simulink model "Differential_polar_nrz"  (R2020b)
settings: Solver=VariableStepAuto  StartTime=0.0  StopTime=20.0  RelTol=1e-3
libraries: commrandsrc3 x1
settings Model: Creator=mluser  LastModifiedBy=mluser

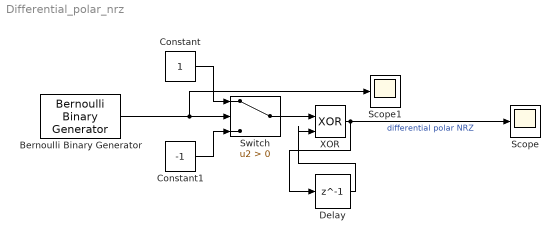
== system Differential_polar_nrz ==
  Bernoulli Binary Generator : commrandsrc3/Bernoulli Binary Generator  ProbabilityOfZero=0.5  SeedSource=Auto  Seed=0  SampleTime=1  SamplesPerFrame=1  OutputDataType=double  SimulateUsing=Interpreted execution
  Constant : Constant
  Constant1 : Constant  Value=-1
  Delay : Delay  DelayLength=1
  Scope : Scope
  Scope1 : Scope
  Switch : Switch  Criteria=u2 > Threshold
  XOR : Logic  Operator=XOR  IconShape=distinctive  AllPortsSameDT=off  OutDataTypeStr=boolean
  wires:
  XOR/1 -> Delay/1, Scope/1  "differential polar NRZ"
  Delay/1 -> XOR/2
  Bernoulli Binary Generator/1 -> Scope1/1, Switch/2
  Switch/1 -> XOR/1
  Constant/1 -> Switch/1
  Constant1/1 -> Switch/3
